simulink model "ConfigurableSS1"  (R2017b)
settings: Solver=FixedStepAuto  StartTime=0.0  StopTime=10.0  FixedStep=1.000000  RelTol=1e-3
settings Model: Creator=hbourbou  LastModifiedBy=hbourbou

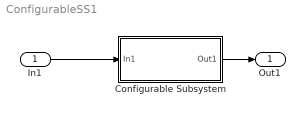
== system ConfigurableSS1 ==
  In1 : Inport
  Configurable Subsystem : Subsystem  BlockChoice=L3
      settings: AttributesFormatString=%<BlockChoice>  MemberBlocks=L1,L2,L3
      settings: TemplateBlock=|
      | library_test/Configurable
      | Subsystem
  Out1 : Outport
  wires:
  In1/1 -> Configurable Subsystem/1(In1)
  Configurable Subsystem/1(Out1) -> Out1/1

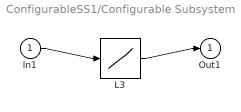
== system ConfigurableSS1/Configurable Subsystem ==
  In1 : Inport
  L3 : Lookup_n-D  NumberOfTableDimensions=1  BreakpointsForDimension1=[-5:5]  Table=sin([-5:5])  InternalRulePriority=Speed  RndMeth=Simplest  InputSameDT=on
  Out1 : Outport
  wires:
  In1/1 -> L3/1
  L3/1 -> Out1/1
